simulink model "atrias_HW_boom_nmSt_kinSw_v2"  (R2015a)
settings: Solver=ode4  StartTime=0.0  StopTime=inf  FixedStep=sample_time  RelTol=1e-3
values from neighbouring files (symbols this model uses):
  control_start_time = 15    [setParams.m]
  flag_CtrlMode = 0    [setParams.m]
  kinSw_alpha_start = 130*pi/180    (= 2.26892802759)    [setParams.m]
  kinSw_alpha_tgt = 70*pi/180    (= 1.2217304764)    [setParams.m]
  kinSw_t_start = 0.5    [setParams.m]
  poser_LLegAlp = (initial_l_leg_angle -pi/2)*180/pi    (= 105)    [setParams.m]
  poser_LLegLen = initial_l_leg_length    (= 0.8)    [setParams.m]
  poser_RLegAlp = (initial_r_leg_angle -pi/2)*180/pi    (= 75)    [setParams.m]
  poser_RLegLen = initial_r_leg_length    (= 0.8)    [setParams.m]
  tune_kinSw_alpha_start = kinSw_alpha_start*180/pi    (= 130)    [setParams.m]
  tune_kinSw_alpha_tgt = kinSw_alpha_tgt*180/pi    (= 70)    [setParams.m]
  tune_kinSw_len_min = kinSw_len_min    (= 0.6)    [setParams.m]
  tune_kinSw_len_tgt = kinSw_len_tgt    (= 0.9)    [setParams.m]
  tune_M1_G = 9.5    [setParams.m]
  tune_M3_0 = CtrlPar_theta0*180/pi    [setParams.m]
  tune_M3_D = St_GainDTh_HFL*5    [setParams.m]
  tune_M3_P = St_GainTh_HFL*5    [setParams.m]
undefined symbols (not defined in the file or in its folder): A1_notch_f1, A2_notch_f1, A_kalman_fourbar_gear, A_lpf_dtau, B1_lpf_dtau, B1_notch_f1, B2_lpf_dtau, B2_notch_f1, B_kalman_fourbar_gear, boom_mount_angle, boom_mount_to_center_diagonal, c_jointstop, C_kalman_fourbar_gear, contactThr, d_vertical_com, delta_phi_max, delta_phi_max_buffer, delta_phi_max_dropoff, delta_phi_min, Discrete, FmaxBFSH, FmaxGLU, FmaxHAM, FmaxHFL, FmaxRF, FmaxVAS, FPCtrlPar, g, gain_nodes_sea_torque, HIP_MTR_MAX_CONT_TORQUE, initial_dx_estimate, j_motor, k_leg_spring, K_notch_f1, k_sea, kalman_load_to_deflect_transmission, kd_lateral, kd_motor, kd_shin_max, kd_shin_min, kd_splay_max, kd_splay_min, kd_thigh_max, kd_thigh_min, kp_lateral, kp_motor, kp_sea_torque, kp_shin_max, kp_shin_min, kp_splay_max, kp_splay_min, kp_thigh_max, kp_thigh_min, l_boom, l_seg, l_v, lateral_motor_efficiency, lateral_offset, lateral_target_angle_right, lateral_transition_force ... (+124)
libraries: simulink_extras x27, simulink x11, ctrlSharedLib x4
(part 8 of 8)

== system atrias_HW_boom_nmSt_kinSw_v2/Control/Behavior Control/Virtual Neuromuscular Control/Torque Distribution/mech limit avoidance1/PD Joint Limit1/R scale desired torque1 ==
  note: NOTE: min_splay_angle does not equal delta_phi_min
  phi_thigh [rad] : Inport
  phi_shin [rad] : Inport  Port=2
  k : Inport  Port=3
  Constant : Constant
  Constant1 : Constant  Value=delta_phi_max - delta_phi_max_buffer
  Constant10 : Constant  Value=phi_thigh_max_buffer
  Constant11 : Constant  Value=phi_shin_min_buffer
  Constant12 : Constant  Value=phi_shin_max_buffer
  Constant13 : Constant
  Constant2 : Constant  Value=phi_thigh_max - phi_thigh_max_buffer
  Constant3 : Constant  Value=min_splay_angle
  Constant4 : Constant  Value=phi_thigh_min + phi_thigh_min_buffer
  Constant5 : Constant  Value=phi_shin_max - phi_shin_max_buffer
  Constant6 : Constant  Value=phi_shin_min + phi_shin_min_buffer
  Constant7 : Constant  Value=min_splay_angle - delta_phi_min
  Constant8 : Constant  Value=delta_phi_max_buffer
  Constant9 : Constant  Value=phi_thigh_min_buffer
  Demux : Demux  Outputs=2
  Divide{,1..5} (6 alike) : Product  Inputs=/*
  Gain : Gain  Gain=-1
  Gain1 : Gain  Gain=-1
  Gain2 : Gain  Gain=-1
  L scale hip/knee : Scope  NumInputPorts=4
      settings: ShowLegends=on  TimeRange=2.5  YMin=-100~-5e+07~-1e+07~-5  YMax=100~1e+07~5e+07~5  SaveName=ScopeData5
  Mux{,3,7..8} (4 alike) : Mux  Inputs=2
  Sum : Sum  Inputs=|+-
  Sum1 : Sum  Inputs=-+|
  Sum2 : Sum  Inputs=+-
  Sum{3..8} (6 alike) : Sum  Inputs=+-|
  [0,1]{,1..6} (7 alike) : Saturate  UpperLimit=1  LowerLimit=0
  max : MinMax  Function=max  Inputs=4
  max1 : MinMax  Function=max  Inputs=4
  to hip_knee : MATLAB Function  TreatAsAtomicUnit=on
  scale_hip : Outport
  scale_knee : Outport  Port=2
  wires:
  "[0,1]6"/1 -> Demux/1
  Mux3/1 -> L scale hip/knee/4
  Demux/2 -> Sum1/1
  Demux/1 -> Sum/2
  to hip_knee/1(scale_hip_knee) -> "[0,1]6"/1
  k/1 -> to hip_knee/3(k)
  max1/1 -> to hip_knee/2(scale_front)
  max/1 -> to hip_knee/1(scale_back)
  Sum1/1 -> scale_knee/1, Mux3/2
  [min_thigh_scale] -> max1/3
  [max_thigh_scale] -> max1/4
  [max_splay_scale] -> max/4, max1/2
  [min_splay_scale] -> max/3, max1/1
  [max_shin_scale] -> max/2
  [min_shin_scale] -> max/1
  Constant13/1 -> Sum1/2
  Gain2/1 -> Divide5/2
  Constant12/1 -> Divide5/1
  Sum7/1 -> Gain2/1
  "[0,1]5"/1 -> [max_shin_scale]
  Divide5/1 -> "[0,1]5"/1
  Constant11/1 -> Divide4/1
  Sum8/1 -> Divide4/2
  "[0,1]4"/1 -> [min_shin_scale]
  Divide4/1 -> "[0,1]4"/1
  Constant10/1 -> Divide3/1
  Sum5/1 -> Gain1/1
  Gain1/1 -> Divide3/2
  "[0,1]3"/1 -> [max_thigh_scale]
  Divide3/1 -> "[0,1]3"/1
  Constant9/1 -> Divide2/1
  Sum6/1 -> Divide2/2
  "[0,1]2"/1 -> [min_thigh_scale]
  Divide2/1 -> "[0,1]2"/1
  Gain/1 -> Divide1/2
  Constant8/1 -> Divide1/1
  Sum3/1 -> Gain/1
  "[0,1]1"/1 -> [max_splay_scale]
  Divide1/1 -> "[0,1]1"/1
  "[0,1]"/1 -> [min_splay_scale]
  Divide/1 -> "[0,1]"/1
  Sum4/1 -> Divide/2
  Constant7/1 -> Divide/1
  Constant/1 -> Sum/1
  Sum/1 -> scale_hip/1, Mux3/1
  [max_splay_scale] -> Mux7/2  "max_splay_trq"
  [min_splay_scale] -> Mux7/1  "min_splay_trq"
  Mux7/1 -> L scale hip/knee/3
  Mux8/1 -> L scale hip/knee/2
  [max_shin_scale] -> Mux8/2  "max_shin_trq"
  [min_shin_scale] -> Mux8/1  "min_shin_trq"
  Mux/1 -> L scale hip/knee/1
  [max_thigh_scale] -> Mux/2  "max_thigh_trq"
  [min_thigh_scale] -> Mux/1  "min_thigh_trq"
  Constant5/1 -> Sum7/1
  [shin] -> Sum7/2
  Constant6/1 -> Sum8/1
  [shin] -> Sum8/2
  Constant2/1 -> Sum5/1
  [thigh] -> Sum5/2
  Constant4/1 -> Sum6/1
  [thigh] -> Sum6/2
  Constant1/1 -> Sum3/1
  [splay] -> Sum3/2
  Constant3/1 -> Sum4/1
  [splay] -> Sum4/2
  Sum2/1 -> [splay]  "splay angle"
  phi_thigh [rad]/1 -> Sum2/2, [thigh]
  phi_shin [rad]/1 -> Sum2/1, [shin]

== matlab function atrias_HW_boom_nmSt_kinSw_v2/Control/Behavior Control/Virtual Neuromuscular Control/Torque Distribution/mech limit avoidance1/PD Joint Limit1/R scale desired torque/to hip_knee ==
  data: scale_back input; scale_hip_knee output; scale_front input; k input
function scale_hip_knee = fcn(scale_back,scale_front,k)

J_inv_trans = [1,1;
               -((k+1)/(2*k)),-((k-1)/(2*k))];
           
scale_hip_knee = J_inv_trans*[scale_back;scale_front];

== matlab function atrias_HW_boom_nmSt_kinSw_v2/Control/Behavior Control/Virtual Neuromuscular Control/Torque Distribution/map_tau_R ==
  settings: updateMethod=DISCRETE  sampleTime=sample_time
  data: tauH_des input; tauB output; tauK_des input; tauF output; k input; Jinv_trans output
function [tauB,tauF, Jinv_trans] = map_virtual_torques(tauH_des,tauK_des,k)
%% FOR REFERENCE: 
%   [dphi_hip; dphi_knee] = J * [dq_back; dq_front];
%   
%   [dq_back; dq_front] = J^(-1) * [dphi_hip; dphi_knee];
%
%   [tauB; tauF] = Jt * [tauH, tauK]
%   
%   [tauH, tauK] = Jt^(-1) * [tauB; tauF]
%
%   J = [(1-k)/2    (1+k)/2 ]   where   k = l_s*sin((q_back-q_front)/2) /
%       [-k         k       ]               l_v*cos(phi_knee/2)
%
% 

%% Construct jacobian, then map virtual torques to actuator torques
j11 = (1-k)/2;
j12 = (1+k)/2;
j21 = -k;
j22 = k;

J = [j11, j12; j21, j22]; 
Jinv_trans = inv(J)';

tau_q = J'*[tauH_des; tauK_des];

tauB = tau_q(1);
tauF = tau_q(2);

end

== matlab function atrias_HW_boom_nmSt_kinSw_v2/Control/Behavior Control/Virtual Neuromuscular Control/Torque Distribution/mech limit avoidance1/PD Joint Limit1/R scale desired torque1/to hip_knee ==
  data: scale_back input; scale_hip_knee output; scale_front input; k input
function scale_hip_knee = fcn(scale_back,scale_front,k)

J_inv_trans = [1,1;
               -((k+1)/(2*k)),-((k-1)/(2*k))];
           
scale_hip_knee = J_inv_trans*[scale_back;scale_front];

== matlab function atrias_HW_boom_nmSt_kinSw_v2/Control/Behavior Control/Virtual Neuromuscular Control/Torque Distribution/map_tau_L ==
  settings: updateMethod=DISCRETE  sampleTime=sample_time
  data: tauH_des input; tauB output; tauK_des input; tauF output; k input; Jinv_trans output
function [tauB,tauF, Jinv_trans] = map_virtual_torques(tauH_des,tauK_des,k)
%% FOR REFERENCE: 
%   [dphi_hip; dphi_knee] = J * [dq_back; dq_front];
%   
%   [dq_back; dq_front] = J^(-1) * [dphi_hip; dphi_knee];
%
%   [tauB; tauF] = Jt * [tauH, tauK]
%   
%   [tauH, tauK] = Jt^(-1) * [tauB; tauF]
%
%   J = [(1-k)/2    (1+k)/2 ]   where   k = l_s*sin((q_back-q_front)/2) /
%       [-k         k       ]               l_v*cos(phi_knee/2)
%
% 

%% Construct jacobian, then map virtual torques to actuator torques
j11 = (1-k)/2;
j12 = (1+k)/2;
j21 = -k;
j22 = k;

J = [j11, j12; j21, j22]; 
Jinv_trans = inv(J)';

tau_q = J'*[tauH_des; tauK_des];

tauB = tau_q(1);
tauF = tau_q(2);

end

== matlab function atrias_HW_boom_nmSt_kinSw_v2/Control/Behavior Control/Virtual Neuromuscular Control/Torque Distribution/mech limit avoidance1/PD Joint Limit1/to hip_knee ==
  data: Rtau_back input; tau_pd_hip_knee output; Rtau_front input; Ltau_back input; Ltau_front input; kR input; kL input
function tau_pd_hip_knee = fcn(Rtau_back,Rtau_front,Ltau_back,Ltau_front,kR,kL)

J_inv_trans = [1,1,0,0;
               -((kR+1)/(2*kR)),-((kR-1)/(2*kR)),0,0;
               0,0,1,1;
               0,0,-((kL+1)/(2*kL)),-((kL-1)/(2*kL))];
           
tau_pd_hip_knee = J_inv_trans*[Rtau_back;
                               Rtau_front;
                               Ltau_back;
                               Ltau_front];

== matlab function atrias_HW_boom_nmSt_kinSw_v2/Control/Behavior Control/Lateral Motor Control/Lateral Control1 ==
  data: tau_r output size=1; qLateralR input; dqLateralR input; qLateralL input; dqLateralL input; F_leg_R input; F_leg_L input; lateral_transition_force parameter; lateral_target_angle_right parameter; m_leg_motor parameter; m_leg parameter; g parameter; lateral_offset parameter; tau_l output size=1; kp_lateral parameter; kd_lateral parameter; minimum_lateral_angle parameter; maximum_lateral_angle parameter; HIP_MTR_MAX_CONT_TORQUE parameter
function [tau_r, tau_l] = LateralBoomControl(...
    qLateralR, dqLateralR, qLateralL, dqLateralL, F_leg_R, F_leg_L,...
    lateral_transition_force, lateral_target_angle_right,...
    m_leg_motor, m_leg, g, lateral_offset,...
    kp_lateral, kd_lateral, minimum_lateral_angle, maximum_lateral_angle, HIP_MTR_MAX_CONT_TORQUE)
    
    % Only add gravity compensation to PD when suspended from winch (approximately static)
    gravity_compensation = 0;
    
    % Inertia for feedforward accelerations
    motor_inertia = (m_leg_motor+m_leg)*lateral_offset^2;
    
    % Right Leg
    right_target = [lateral_target_angle_right, 0, 0];
    desired = [saturate(right_target(1),minimum_lateral_angle,maximum_lateral_angle), right_target(2)];
    measured = [qLateralR, dqLateralR];
    tau_r = [kp_lateral, kd_lateral] * (desired-measured)' + gravity_compensation + motor_inertia*right_target(3);
    tau_r = max(min(HIP_MTR_MAX_CONT_TORQUE, tau_r),-HIP_MTR_MAX_CONT_TORQUE);
    
    if (F_leg_R >= lateral_transition_force)
        tau_r = -lateral_offset*(F_leg_R-(m_leg_motor+m_leg)*g);
    end
    
    % Left Leg
    left_target = [lateral_target_angle_right, 0, 0];
    desired = [saturate(left_target(1),minimum_lateral_angle,maximum_lateral_angle), left_target(2)];
    measured = [qLateralL, dqLateralL];
    tau_l = [kp_lateral, kd_lateral] * (desired-measured)' + gravity_compensation + motor_inertia*left_target(3);
    tau_l = max(min(HIP_MTR_MAX_CONT_TORQUE, tau_l),-HIP_MTR_MAX_CONT_TORQUE);
    
    if (F_leg_L >= lateral_transition_force)
        tau_l = -lateral_offset*(F_leg_L-(m_leg_motor+m_leg)*g);
    end
end

function [desired_saturated] = saturate(desired, minimum_lateral_angle, maximum_lateral_angle)
    desired_saturated = desired;
    if desired(1) < minimum_lateral_angle
        desired_saturated = [minimum_lateral_angle, 0];
    elseif desired(1) > maximum_lateral_angle
        desired_saturated = [maximum_lateral_angle, 0];    
    end
end

== matlab function atrias_HW_boom_nmSt_kinSw_v2/Control/Behavior Control/kinematic swing leg controller/Avoid Hitting Mechanical Limits ==
  data: back_cmd output double; front_cmd output double; dback_cmd output double; dfront_cmd output double; ddback_cmd output double; ddfront_cmd output double; back_desired input; dback_desired input; ddback_desired input; front_desired input; dfront_desired input; ddfront_desired input; min_front_bar_angle input; max_front_bar_angle input; min_back_bar_angle input; max_back_bar_angle input
%% Avoid joint limits by ensuring we don't command velocities/accelerations that would push us into them when we are close to them.
function [back_cmd, front_cmd, dback_cmd, dfront_cmd, ddback_cmd, ddfront_cmd] ...
    = AvoidFourbarLimits(back_desired,dback_desired, ddback_desired, ...
          front_desired, dfront_desired, ddfront_desired, ...
          min_front_bar_angle, max_front_bar_angle, min_back_bar_angle, max_back_bar_angle)
    [back_cmd, front_cmd, dback_cmd, dfront_cmd, ddback_cmd, ddfront_cmd] = AvoidFourbarLimits(back_desired,dback_desired, ddback_desired, front_desired, dfront_desired, ddfront_desired, min_front_bar_angle, max_front_bar_angle, min_back_bar_angle, max_back_bar_angle);
end

== matlab function atrias_HW_boom_nmSt_kinSw_v2/Control/Poser/Subsystem/Avoid Hitting Mechanical Limits ==
  data: back_cmd output double; front_cmd output double; dback_cmd output double; dfront_cmd output double; ddback_cmd output double; ddfront_cmd output double; back_desired input; dback_desired input; ddback_desired input; front_desired input; dfront_desired input; ddfront_desired input; min_front_bar_angle input; max_front_bar_angle input; min_back_bar_angle input; max_back_bar_angle input
%% Avoid joint limits by ensuring we don't command velocities/accelerations that would push us into them when we are close to them.
function [back_cmd, front_cmd, dback_cmd, dfront_cmd, ddback_cmd, ddfront_cmd] ...
    = AvoidFourbarLimits(back_desired,dback_desired, ddback_desired, ...
          front_desired, dfront_desired, ddfront_desired, ...
          min_front_bar_angle, max_front_bar_angle, min_back_bar_angle, max_back_bar_angle)
    [back_cmd, front_cmd, dback_cmd, dfront_cmd, ddback_cmd, ddfront_cmd] = AvoidFourbarLimits(back_desired,dback_desired, ddback_desired, front_desired, dfront_desired, ddfront_desired, min_front_bar_angle, max_front_bar_angle, min_back_bar_angle, max_back_bar_angle);
end

== matlab function atrias_HW_boom_nmSt_kinSw_v2/Control/Behavior Control/kinematic swing leg controller/Generate Parabolic Leg Trajectories ==
  data: legLen_ref output size=3; flight input; legLen0 input; legLen_clr input; legLen_star input; alpha_start input; alpha_star input; alpha input
%% Parabolic trajectory generation for leg angle and length
% est_duration: estimated flight time
% time_remaining: time until estimated touchdown
% legAlp0: legAlp at takeoff
%   legAlp is the angle of attack
% legLen0: legLen at takeoff
% legAlp_star: desired legAlp
% legLen_star: desired legLen
% legLen_min: min legLen for ground clearance
% min_f_duration: minimum trajectory time

function legLen_ref   =  ...
          GenerateReferenceLegLength(flight, ...
                    legLen0, legLen_clr, legLen_star,   ...
                    alpha_start, alpha_star, alpha)

if ~flight
    legLen_ref = [0.9;0;0];
    return;
end

    
  % split duration into thirds.  First segment: parabola from legLen0 to
  % legLen_min.  Second and third segments, cos to landing.
  alpha_d   = abs(alpha_star-alpha_start);
  alpha_r   = max(abs(alpha_star-alpha), 0);
  da3 = alpha_d / 3;
  if alpha_r > 2*da3;
    legLen_star_a = legLen_clr + (legLen0-legLen_clr)*((alpha_r-2*da3)/da3)^2;
    dlegLen_star_a = -(legLen0-legLen_clr)*2*(alpha_r-2*da3)/da3/da3;
    ddlegLen_star_a = (legLen0-legLen_clr)*2/da3^2;
  else
    legLen_star_a = legLen_star + (legLen_clr-legLen_star)/2*(1-cos(alpha_r/(2*da3)*pi));
    dlegLen_star_a = -(legLen_clr-legLen_star)/2*sin(alpha_r/(2*da3)*pi)*pi/(2*da3);
    ddlegLen_star_a = (legLen_clr-legLen_star)/2*cos(alpha_r/(2*da3)*pi)*(pi/(2*da3))^2;
  end
  
  % track a sinusoidal z of amplitude max_retract, finishing a half-cycle by t_end
  legLen_ref = [legLen_star_a; dlegLen_star_a; ddlegLen_star_a];

== matlab function atrias_HW_boom_nmSt_kinSw_v2/Control/Poser/Subsystem/Avoid Hitting Mechanical Limits1 ==
  data: back_cmd output double; front_cmd output double; dback_cmd output double; dfront_cmd output double; ddback_cmd output double; ddfront_cmd output double; back_desired input; dback_desired input; ddback_desired input; front_desired input; dfront_desired input; ddfront_desired input; min_front_bar_angle input; max_front_bar_angle input; min_back_bar_angle input; max_back_bar_angle input
%% Avoid joint limits by ensuring we don't command velocities/accelerations that would push us into them when we are close to them.
function [back_cmd, front_cmd, dback_cmd, dfront_cmd, ddback_cmd, ddfront_cmd] ...
    = AvoidFourbarLimits(back_desired,dback_desired, ddback_desired, ...
          front_desired, dfront_desired, ddfront_desired, ...
          min_front_bar_angle, max_front_bar_angle, min_back_bar_angle, max_back_bar_angle)
    [back_cmd, front_cmd, dback_cmd, dfront_cmd, ddback_cmd, ddfront_cmd] = AvoidFourbarLimits(back_desired,dback_desired, ddback_desired, front_desired, dfront_desired, ddfront_desired, min_front_bar_angle, max_front_bar_angle, min_back_bar_angle, max_back_bar_angle);
end

== matlab function atrias_HW_boom_nmSt_kinSw_v2/Control/Poser/Subsystem/Virtual Leg to Four Bar ==
  data: l_leg input; dl_leg input; ddl_leg input; phi input; dphi input; ddphi input; back output; dback output; ddback output; front output; dfront output; ddfront output
function [back, dback, ddback, front, dfront, ddfront] = VirtualLegToFourBar(l_leg, dl_leg, ddl_leg, phi, dphi, ddphi)
    [back, dback, ddback, front, dfront, ddfront] = VirtualLegToFourBar(l_leg, dl_leg, ddl_leg, phi, dphi, ddphi);
end

== matlab function atrias_HW_boom_nmSt_kinSw_v2/Control/Behavior Control/kinematic swing leg controller/Virtual Leg to Four Bar ==
  data: l_leg input; dl_leg input; ddl_leg input; phi input; dphi input; ddphi input; back output; dback output; ddback output; front output; dfront output; ddfront output
function [back, dback, ddback, front, dfront, ddfront] = VirtualLegToFourBar(l_leg, dl_leg, ddl_leg, phi, dphi, ddphi)
    [back, dback, ddback, front, dfront, ddfront] = VirtualLegToFourBar(l_leg, dl_leg, ddl_leg, phi, dphi, ddphi);
end

== matlab function atrias_HW_boom_nmSt_kinSw_v2/Control/Poser/Subsystem/Virtual Leg to Four Bar1 ==
  data: l_leg input; dl_leg input; ddl_leg input; phi input; dphi input; ddphi input; back output; dback output; ddback output; front output; dfront output; ddfront output
function [back, dback, ddback, front, dfront, ddfront] = VirtualLegToFourBar(l_leg, dl_leg, ddl_leg, phi, dphi, ddphi)
    [back, dback, ddback, front, dfront, ddfront] = VirtualLegToFourBar(l_leg, dl_leg, ddl_leg, phi, dphi, ddphi);
end

== matlab function atrias_HW_boom_nmSt_kinSw_v2/Fourbar Gearside Kalman Filter/External Trunk Torque Estimate ==
  data: grf_xz input; rotor_torque input; spring_torque input; tau_trunk output; torso_pitch input; d_vertical_com parameter; LEG_MTR_GEAR_RATIO parameter
function tau_trunk = tau_trunk(grf_xz, rotor_torque, spring_torque, torso_pitch, d_vertical_com, LEG_MTR_GEAR_RATIO )
    d = d_vertical_com;
    theta = torso_pitch;
    N = LEG_MTR_GEAR_RATIO;
    tau_trunk = sum(-rotor_torque + -(N-1)/N*spring_torque) + (-d*cos(theta)*grf_xz(1) + d*sin(theta)*grf_xz(2));
end

== matlab function atrias_HW_boom_nmSt_kinSw_v2/Fourbar Gearside Kalman Filter/Covariance Estimates ==
  data: spring_torque input; absolute_gear input; current_position_estimate input; state_uncertainty input; Q1 output; R1 output; Q2 output; R2 output; R_kalman_absolute_normal parameter; R_kalman_absolute_fail parameter; R_kalman_incremental_unloaded parameter; R_kalman_incremental_loaded parameter; kalman_load_to_deflect_transmission parameter; Q3 output; R3 output; Q4 output; R4 output; max_absolute_measurement_innovation parameter; k_sea parameter; Q_kalman_spring_torque parameter; Q_kalman_rotor_torque parameter; Q_kalman_trunk_torque parameter; sample_time parameter
function [Q1, R1, Q2, R2, Q3, R3, Q4, R4] = covariance( spring_torque, absolute_gear, current_position_estimate, state_uncertainty, R_kalman_absolute_normal, R_kalman_absolute_fail, R_kalman_incremental_unloaded, R_kalman_incremental_loaded, kalman_load_to_deflect_transmission, max_absolute_measurement_innovation, k_sea, Q_kalman_spring_torque, Q_kalman_rotor_torque, Q_kalman_trunk_torque, sample_time)

    persistent previous_absolute_gear
    if isempty(previous_absolute_gear)
        previous_absolute_gear = absolute_gear;
    end
    
    % Measurement covariance
    R_absolute = ones(4,1)*R_kalman_absolute_normal;
    dropped_out = previous_absolute_gear == absolute_gear;
    out_of_range = abs(current_position_estimate - absolute_gear) > max_absolute_measurement_innovation;
    R_absolute(dropped_out | out_of_range) = R_kalman_absolute_fail;
    
    R_incremental_scale = min(abs(spring_torque)/kalman_load_to_deflect_transmission, 1);
    R_incremental = R_incremental_scale*R_kalman_incremental_loaded + (1-R_incremental_scale)*R_kalman_incremental_unloaded;
    
    R1 = diag([R_absolute(1), R_incremental(1)])/sample_time;
    R2 = diag([R_absolute(2), R_incremental(2)])/sample_time;
    R3 = diag([R_absolute(3), R_incremental(3)])/sample_time;
    R4 = diag([R_absolute(4), R_incremental(4)])/sample_time;
    
    % Process noise covariance
    Q_spring_torque = k_sea'.^2.*(state_uncertainty + R_kalman_absolute_normal) + Q_kalman_spring_torque;

    Q1 = diag([Q_spring_torque(1), Q_kalman_rotor_torque, Q_kalman_trunk_torque]);
    Q2 = diag([Q_spring_torque(2), Q_kalman_rotor_torque, Q_kalman_trunk_torque]);
    Q3 = diag([Q_spring_torque(3), Q_kalman_rotor_torque, Q_kalman_trunk_torque]);
    Q4 = diag([Q_spring_torque(4), Q_kalman_rotor_torque, Q_kalman_trunk_torque]);

    previous_absolute_gear = absolute_gear;
end

== matlab function atrias_HW_boom_nmSt_kinSw_v2/Fourbar Gearside Kalman Filter/eigen values 1 ==
  data: Z input; E output
function E = eigen(Z)
    E = real(eig(Z));
    E = sort(E);
end

== matlab function atrias_HW_boom_nmSt_kinSw_v2/Fourbar Gearside Kalman Filter/eigen values 2 ==
  data: Z input; E output
function E = eigen(Z)
    E = real(eig(Z));
    E = sort(E);
end

== matlab function atrias_HW_boom_nmSt_kinSw_v2/Fourbar Gearside Kalman Filter/eigen values 3 ==
  data: Z input; E output
function E = eigen(Z)
    E = real(eig(Z));
    E = sort(E);
end

== matlab function atrias_HW_boom_nmSt_kinSw_v2/Fourbar Gearside Kalman Filter/eigen values4  ==
  data: Z input; E output
function E = eigen(Z)
    E = real(eig(Z));
    E = sort(E);
end
